simulink model "JKFF2"  (R2025a)
settings: Solver=VariableStepAuto  StartTime=0.0  StopTime=inf  RelTol=1e-3
libraries: simulink_extras x1
settings Model: Creator=Soochan Kim  LastModifiedBy=Soochan Kim

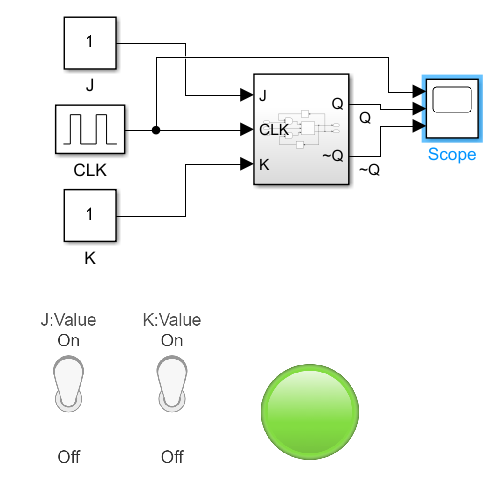
[thumbnail: Simulink's stored preview of the top-level diagram]
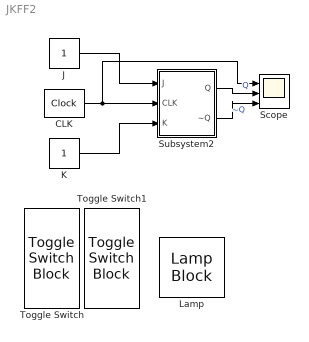
== system JKFF2 ==
  CLK : simulink_extras/Flip Flops/Clock  period=0.5
  J : Constant
  K : Constant
  Lamp : LampBlock  LabelPosition=Hide  DefaultColor=[192.0, 192.0, 192.0]
  Scope : Scope  NumInputPorts=3
      settings: ActiveDisplayYMinimum=-0.12499999999999997  ActiveDisplayYMaximum=1.125
  Subsystem2 : Subsystem
  Toggle Switch : ToggleSwitchBlock
  Toggle Switch1 : ToggleSwitchBlock
  wires:
  CLK/1 -> Scope/1, Subsystem2/2(CLK)
  Subsystem2/1(Q) -> Scope/2  "Q"
  Subsystem2/2(~Q) -> Scope/3  "~Q"
  J/1 -> Subsystem2/1(J)
  K/1 -> Subsystem2/3(K)

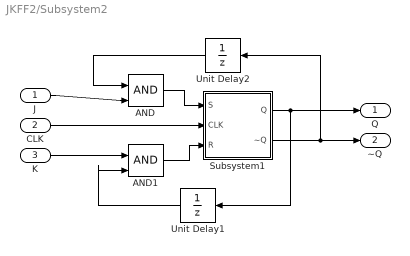
== system JKFF2/Subsystem2 ==
  J : Inport
  CLK : Inport  Port=2
  K : Inport  Port=3
  AND : Logic  IconShape=distinctive  AllPortsSameDT=off  OutDataTypeStr=boolean
  AND1 : Logic  IconShape=distinctive  AllPortsSameDT=off  OutDataTypeStr=boolean
  Subsystem1 : Subsystem
  Unit Delay1 : UnitDelay  SampleTime=-1  HasFrameUpgradeWarning=on
  Unit Delay2 : UnitDelay  SampleTime=-1  HasFrameUpgradeWarning=on
  Q : Outport
  ~Q : Outport  Port=2
  wires:
  Unit Delay1/1 -> AND1/2
  Subsystem1/2(~Q) -> Unit Delay2/1, ~Q/1
  AND1/1 -> Subsystem1/3(R)
  AND/1 -> Subsystem1/1(S)
  CLK/1 -> Subsystem1/2(CLK)
  K/1 -> AND1/1
  J/1 -> AND/2
  Subsystem1/1(Q) -> Unit Delay1/1, Q/1
  Unit Delay2/1 -> AND/1

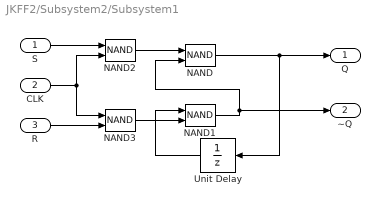
== system JKFF2/Subsystem2/Subsystem1 ==
  S : Inport
  CLK : Inport  Port=2
  R : Inport  Port=3
  NAND{,1..3} (4 alike) : Logic  Operator=NAND  IconShape=distinctive  AllPortsSameDT=off  OutDataTypeStr=boolean
  Unit Delay : UnitDelay  SampleTime=-1  HasFrameUpgradeWarning=on
  Q : Outport
  ~Q : Outport  Port=2
  wires:
  CLK/1 -> NAND2/2, NAND3/1
  NAND1/1 -> NAND/2, ~Q/1
  S/1 -> NAND2/1
  NAND2/1 -> NAND/1
  NAND3/1 -> NAND1/2
  R/1 -> NAND3/2
  NAND/1 -> Q/1, Unit Delay/1
  Unit Delay/1 -> NAND1/1
